simulink model "GoToGoal"  (R2023b)
settings: Solver=VariableStepAuto  StartTime=0.0  StopTime=50.0  RelTol=1e-3
settings Model: Creator=haluk  LastModifiedBy=Baki
settings DebuggingCC: UnconnectedInputMsg=warning  UnconnectedOutputMsg=warning  UnconnectedLineMsg=warning
settings ModelReferenceCC: EnableRefExpFcnMdlSchedulingChecks=on
settings RTWCC: DLArmComputeVersion=19.05

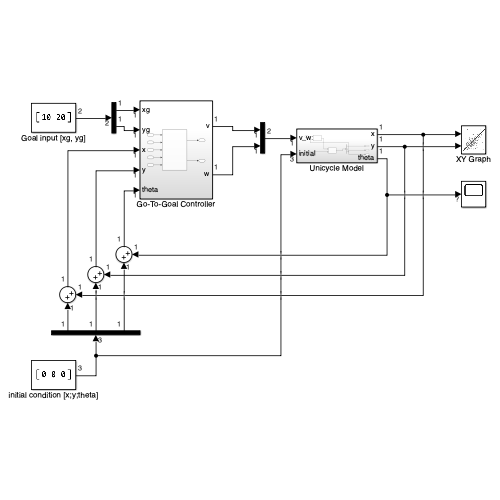
[thumbnail: Simulink's stored preview of the top-level diagram]
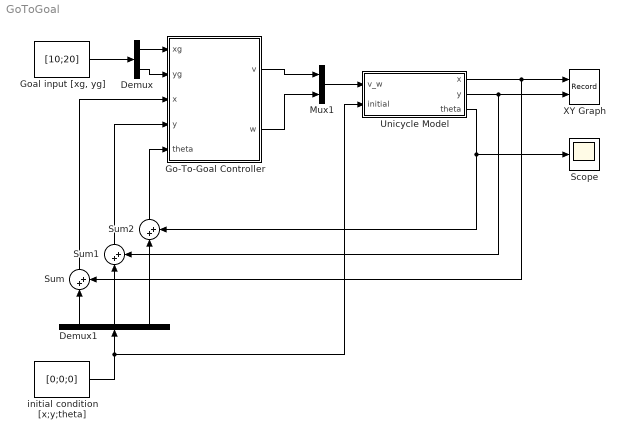
== system GoToGoal ==
  Demux : Demux  Outputs=2
  Demux1 : Demux  Outputs=3
  Go-To-Goal Controller : Subsystem
  "Goal input [xg, yg]" : Constant  Value=[10;20]
  Mux1 : Mux  Inputs=2
  Scope : Scope
  Sum : Sum  Inputs=|++
  Sum1 : Sum  Inputs=|++
  Sum2 : Sum  Inputs=|++
  Unicycle Model : Subsystem
  XY Graph : Record  FileSettingsInternal="{\"entries\":[{\"content\":{\"excelSettings\":{\"content\":{},\"type\":\"Streamout.ExcelSettings\"}},\"type\":\"Streamout.FileSettingStorage\",\"uuid\":\"\"}],\"packageUris\":[\"http:\\/\\/schema.mathworks.com\\/mf0\\/streamout_blocks\\/R2020a\"],\"version\":\"1.0\"}"  Layout=[1 1]  SignalsInternal="{\"entries\":[{\"content\":{\"signals\":[{\"content\":{\"blockPath\":[],\"dimensions\":[1],\"domain\":\"\",\"lineColor\":\"#a2142f\",\"plots\":[1],\"port\":1,\"signalID\":47,\"signalName\":\"XY Graph:1\"},\"type\":\"RecordBlkView.Signal\",\"uuid\":\"\"},{\"content\":{\"blockPath\":[],\"dimensions\":[1],\"domain\":\"\",\"lineColor\":\"#139fff\",\"plots\":[1],\"port\":2,\"signalID\":50,\"signalName\":\"XY Graph:2\"},\"type\":\"RecordBlkView.Signal\",\"uuid\":\"\"}]},\"type\":\"RecordBlkView.InputSignals\",\"uuid\":\"\"}],\"packageUris\":[\"http:\\/\\/schema.mathworks.com\\/mf0\\/streamout_blocks\\/R2020a\"],\"version\":\"1.0\"}"  VisualizationBindings="{\"xyplotplugin\":{\"info\":[{\"series\":[{\"bindingParametersList\":[{\"parameter\":\"X-Axis\",\"signalID\":47,\"signalName\":\"XY Graph:1\"},{\"parameter\":\"Y-Axis\",\"signalID\":50,\"signalName\":\"XY Graph:2\"}],\"seriesID\":8183}],\"subplotID\":1}]}}"  CompatibilityTag=XY  st=-1
  initial condition [x;y;theta] : Constant  Value=[0;0;0]
  wires:
  Unicycle Model/1(x) -> Sum/2, XY Graph/1
  Unicycle Model/2(y) -> Sum1/2, XY Graph/2
  Unicycle Model/3(theta) -> Scope/1, Sum2/2
  Mux1/1 -> Unicycle Model/1(v_w)
  "Goal input [xg, yg]"/1 -> Demux/1
  Demux/1 -> Go-To-Goal Controller/1(xg)
  Demux/2 -> Go-To-Goal Controller/2(yg)
  initial condition [x;y;theta]/1 -> Unicycle Model/2(initial), Demux1/1
  Go-To-Goal Controller/1(v) -> Mux1/1
  Go-To-Goal Controller/2(w) -> Mux1/2
  Demux1/1 -> Sum/1
  Demux1/2 -> Sum1/1
  Demux1/3 -> Sum2/1
  Sum2/1 -> Go-To-Goal Controller/5(theta)
  Sum1/1 -> Go-To-Goal Controller/4(y)
  Sum/1 -> Go-To-Goal Controller/3(x)

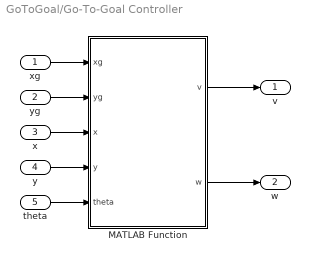
== system GoToGoal/Go-To-Goal Controller ==
  xg : Inport
  yg : Inport  Port=2
  x : Inport  Port=3
  y : Inport  Port=4
  theta : Inport  Port=5
  MATLAB Function : MATLAB Function  TreatAsAtomicUnit=on
  v : Outport
  w : Outport  Port=2
  wires:
  theta/1 -> MATLAB Function/5(theta)
  y/1 -> MATLAB Function/4(y)
  x/1 -> MATLAB Function/3(x)
  yg/1 -> MATLAB Function/2(yg)
  xg/1 -> MATLAB Function/1(xg)
  MATLAB Function/1(v) -> v/1
  MATLAB Function/2(w) -> w/1

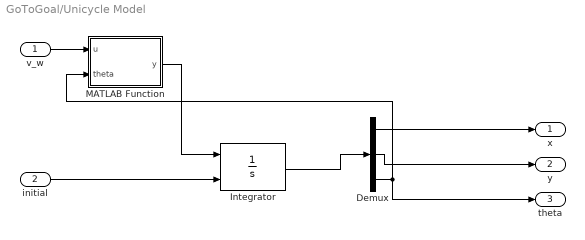
== system GoToGoal/Unicycle Model ==
  v_w : Inport
  initial : Inport  Port=2
  Demux : Demux  Outputs=3
  Integrator : Integrator  InitialConditionSource=external
  MATLAB Function : MATLAB Function  TreatAsAtomicUnit=on
  x : Outport
  y : Outport  Port=2
  theta : Outport  Port=3
  wires:
  MATLAB Function/1(y) -> Integrator/1
  Demux/3 -> theta/1, MATLAB Function/2(theta)
  Integrator/1 -> Demux/1
  Demux/1 -> x/1
  initial/1 -> Integrator/2
  v_w/1 -> MATLAB Function/1(u)
  Demux/2 -> y/1

== matlab function GoToGoal/Unicycle Model/MATLAB Function ==
  data: u input; y output; theta input
function y = fcn(u, theta)


v = u(1);
w = u(2);

y = [v*cos(theta); v*sin(theta); w];

== matlab function GoToGoal/Go-To-Goal Controller/MATLAB Function ==
  data: xg input; yg input; x input; y input; v output; theta input; w output
function [v,w]= fcn(xg,yg,x,y,theta)

Kp = 1.0;
Kh = 1.0;

delta_x = xg - x;
delta_y = yg - y;
theta_g = atan2(delta_y, delta_x);
delta_theta = theta_g - theta;
delta_theta = atan2(sin(delta_theta), cos(delta_theta)); %[-π, π]
uzaklik = sqrt(delta_x^2 + delta_y^2);

% Hız ve dönüş açısı hesaplama
vt = Kp * uzaklik;
wt = Kh * delta_theta;

% Hızı sınırla
if vt > 1
    vt = 1;
end
if wt > pi/4
    wt = pi/4;
end

v = vt;
w = wt;
